simulink model "MS_PID_Control_model"  (R2023a)
settings: Solver=VariableStepAuto  StartTime=0.0  StopTime=2  RelTol=1e-3
values from neighbouring files (symbols this model uses):
  A = [0      1       0           0 ... (first row only)    [MS_PID_Control.m]    (also in SS_PID_Control.m = [0 1;-k/m -c/m])
  amp = 0.01    [MS_PID_Control.m]    (also in SS_PID_Control.m)
  B = [0 k_m/m1 0 -k_m/m2]'    [MS_PID_Control.m]    (also in SS_PID_Control.m = [0;k_f/m])
  C = [-k1/m1 -c1/m1   k1/m1       c1/m1 ... (first row only)    [MS_PID_Control.m]    (also in SS_PID_Control.m = [1 0])
  D = 0    [MS_PID_Control.m]    (also in SS_PID_Control.m)
  den = [L R_m]    [MS_PID_Control.m]
  E = [0 0 0 c2/m2 ... (first row only)    [MS_PID_Control.m]    (also in SS_PID_Control.m = [0 0;c/m k/m])
  Kd = 00070    (= 70)    [MS_PID_Control.m]    (also in SS_PID_Control.m)
  Ki = 13000    [MS_PID_Control.m]    (also in SS_PID_Control.m)
  Kp = 27000    [MS_PID_Control.m]    (also in SS_PID_Control.m)
  num = 1    [MS_PID_Control.m]
libraries: slpidlib x1
settings Model: Creator=z'k'x  LastModifiedBy=z'k'x

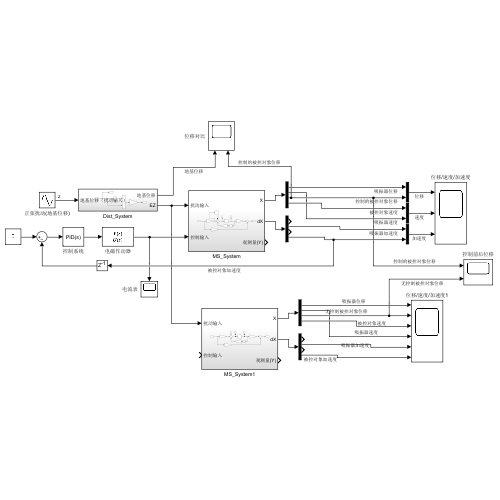
[thumbnail: Simulink's stored preview of the top-level diagram]
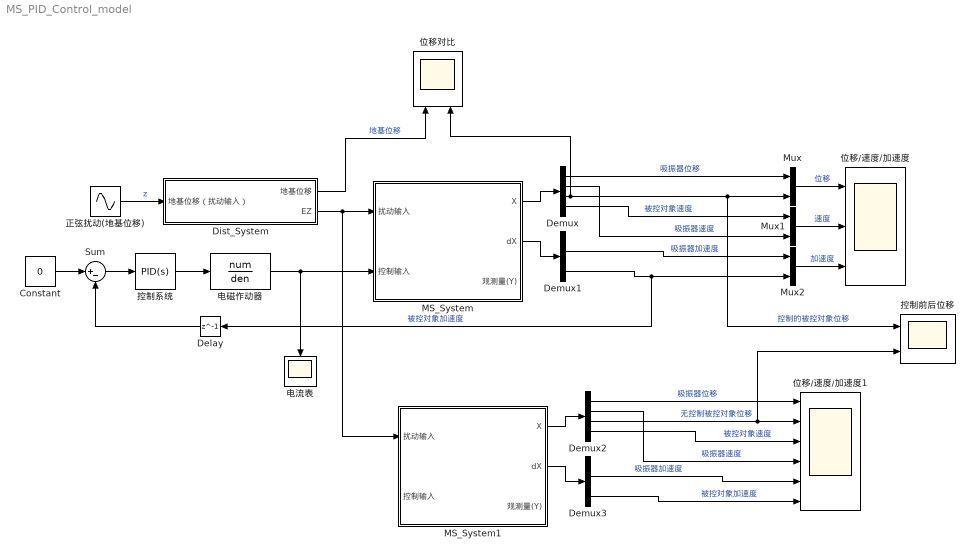
== system MS_PID_Control_model ==
  Constant : Constant  Value=0
  Delay : Delay  DelayLength=1  InitialCondition=0
  Demux{,1..3} (4 alike) : Demux
  Dist_System : Subsystem
  MS_System : Subsystem
  MS_System1 : Subsystem
  Mux : Mux  Inputs=2
  Mux1 : Mux  Inputs=2
  Mux2 : Mux  Inputs=2
  Sum : Sum  Inputs=|+-
  位移/速度/加速度 : Scope  NumInputPorts=3
  位移/速度/加速度1 : Scope  NumInputPorts=6
  位移对比 : Scope  NumInputPorts=2
  控制前后位移 : Scope  NumInputPorts=2
  控制系统 : slpidlib/PID Controller  Controller=PID  Form=Parallel  TimeDomain=Continuous-time  UseExternalTs=off  SampleTime=-1  IntegratorMethod=Forward Euler  FilterMethod=Forward Euler  ControllerParametersSource=internal  P=Kp  I=Ki  UseKiTs=off  D=Kd  N=100  UseFilter=on  TunerSelectOption=Transfer Function Based (PID Tuner App)  InitialConditionSource=internal  InitialConditionForIntegrator=0  InitialConditionForFilter=0  DifferentiatorICPrevScaledInput=0  ExternalReset=none  TrackingMode=off  Kt=1  LimitOutput=off  SatLimitsSource=internal  UpperSaturationLimit=inf  LowerSaturationLimit=-inf  LinearizeAsGain=on  AntiWindupMode=none  Kb=1  LimitIntegrator=off  UpperIntegratorSaturationLimit=inf  LowerIntegratorSaturationLimit=-inf  POutMin=[]  POutMax=[]  IOutMin=[]  IOutMax=[]  DOutMin=[]  DOutMax=[]  NOutMin=[]  NOutMax=[]  SumOutMin=[]  SumOutMax=[]  SaturationOutMin=[]  SaturationOutMax=[]  PParamMin=[]  PParamMax=[]  IParamMin=[]  IParamMax=[]  DParamMin=[]  DParamMax=[]  NParamMin=[]  NParamMax=[]  KbParamMin=[]  KbParamMax=[]  KtParamMin=[]  KtParamMax=[]  KbOutMin=[]  KbOutMax=[]  KtOutMin=[]  KtOutMax=[]  IntegratorOutMin=[]  IntegratorOutMax=[]  FilterOutMin=[]  FilterOutMax=[]  SumI1OutMin=[]  SumI1OutMax=[]  SumI2OutMin=[]  SumI2OutMax=[]  SumI3OutMin=[]  SumI3OutMax=[]  SumI4OutMin=[]  SumI4OutMax=[]  SumDOutMin=[]  SumDOutMax=[]  DifferentiatorOutMin=[]  DifferentiatorOutMax=[]  FilterDiffOutCoefMin=[]  FilterDiffOutCoefMax=[]  ReciprocalOutMin=[]  ReciprocalOutMax=[]  SumDenOutMin=[]  SumDenOutMax=[]  SumNumOutMin=[]  SumNumOutMax=[]  DivideOutMin=[]  DivideOutMax=[]  UdiffTsProdOutMin=[]  UdiffTsProdOutMax=[]  NTsProdOutMin=[]  NTsProdOutMax=[]  UintegralTsProdOutMin=[]  UintegralTsProdOutMax=[]  UngainTsProdOutMin=[]  UngainTsProdOutMax=[]  ClampingZeroOutDataTypeStr=Inherit: Inherit via back propagation  ClampingZeroOutMin=[]  ClampingZeroOutMax=[]  FilterDenConstantOutDataTypeStr=Inherit: Inherit via back propagation  FilterDenConstantOutMin=[]  FilterDenConstantOutMax=[]  PCopyOutDataTypeStr=Inherit: Inherit via back propagation  PCopyOutMin=[]  PCopyOutMax=[]  NCopyOutDataTypeStr=Inherit: Inherit via back propagation  NCopyOutMin=[]  NCopyOutMax=[]  IntegratorContinuousStateAttributes=''  IntegratorStateMustResolveToSignalObject=off  IntegratorRTWStateStorageClass=Auto  FilterContinuousStateAttributes=''  FilterStateMustResolveToSignalObject=off  FilterRTWStateStorageClass=Auto  ParallelPVariant=InternalParameters  IdealPVariant=Disabled  IVariant=InternalParameters  DVariant=InternalParameters  IntegratorVariant=Continuous  SatVariant=Disabled  AWVariant=Passthrough  PCopyVariant=Disabled  TRVariant=Disabled  FdbkBlocksVariant=Forward  IdealPFdbkVariant=Disabled  SatFdbkVariant=Disabled  DerivativeFilterVariant=ContFilter  NVariant=InternalParameters  NCopyVariant=Disabled  FilterICVariant=InternalICsFilter  IntegratorICVariant=InternalICs  ExternalResetVariant=Disabled  TRSumVariant=Passthrough  SumFdbkVariant=Disabled  SumVariant=Sum_PID  TsampFilterVariant=InternalTs  TsampNgainVariant=Passthrough  TsampIntegralVariant=Disabled_SignalSpec  ExternalSaturationOutDataTypeStr=Inherit: Same as second input
  正弦扰动(地基位移) : Sin  Amplitude=amp  Frequency=60*pi  SampleTime=0
  电流表 : Scope
  电磁作动器 : TransferFcn  Numerator=num  Denominator=den
  wires:
  控制系统/1 -> 电磁作动器/1
  正弦扰动(地基位移)/1 -> Dist_System/1(地基位移（扰动输入）)  "z"
  Dist_System/2(EZ) -> MS_System1/1(扰动输入), MS_System/1(扰动输入)
  Dist_System/1(地基位移) -> 位移对比/1  "地基位移"
  MS_System/1(X) -> Demux/1
  MS_System/2(dX) -> Demux1/1
  Demux/1 -> Mux/1  "吸振器位移"
  Demux/4 -> Mux1/1  "被控对象速度"
  Demux/3 -> 位移对比/2, 控制前后位移/1, Mux/2  "控制的被控对象位移"
  Demux/2 -> Mux1/2  "吸振器速度"
  Demux1/2 -> Mux2/1  "吸振器加速度"
  Demux1/4 -> Delay/1, Mux2/2  "被控对象加速度"
  Sum/1 -> 控制系统/1
  Constant/1 -> Sum/1
  Demux3/4 -> 位移/速度/加速度1/6  "被控对象加速度"
  Demux2/3 -> 控制前后位移/2, 位移/速度/加速度1/2  "无控制被控对象位移"
  MS_System1/1(X) -> Demux2/1
  Demux2/4 -> 位移/速度/加速度1/3  "被控对象速度"
  MS_System1/2(dX) -> Demux3/1
  Demux2/2 -> 位移/速度/加速度1/4  "吸振器速度"
  Demux2/1 -> 位移/速度/加速度1/1  "吸振器位移"
  Demux3/2 -> 位移/速度/加速度1/5  "吸振器加速度"
  电磁作动器/1 -> 电流表/1, MS_System/2(控制输入)
  Mux/1 -> 位移/速度/加速度/1  "位移"
  Mux1/1 -> 位移/速度/加速度/2  "速度"
  Mux2/1 -> 位移/速度/加速度/3  "加速度"
  Delay/1 -> Sum/2

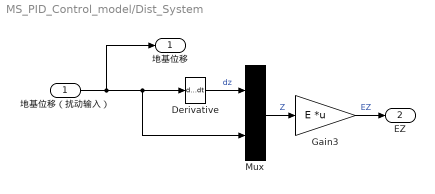
== system MS_PID_Control_model/Dist_System ==
  地基位移（扰动输入） : Inport
  Derivative : Derivative
  Gain3 : Gain  Gain=E  Multiplication=Matrix(K*u) (u vector)
  Mux : Mux  Inputs=2
      settings: DisplayOption=signals
  地基位移 : Outport
  EZ : Outport  Port=2
  wires:
  Gain3/1 -> EZ/1  "EZ"
  Mux/1 -> Gain3/1  "Z"
  Derivative/1 -> Mux/1  "dz"
  地基位移（扰动输入）/1 -> 地基位移/1, Derivative/1, Mux/2

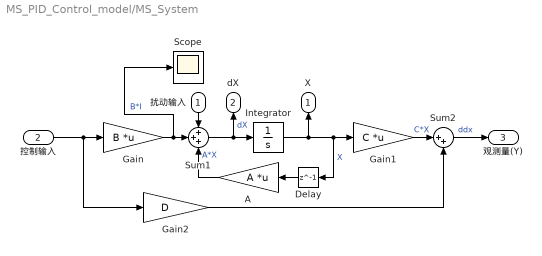
== system MS_PID_Control_model/MS_System ==
  扰动输入 : Inport
  控制输入 : Inport  Port=2
  A : Gain  Gain=A  Multiplication=Matrix(K*u) (u vector)
  Delay : Delay  DelayLength=1  InitialCondition=0
  Gain : Gain  Gain=B  Multiplication=Matrix(K*u) (u vector)
  Gain1 : Gain  Gain=C  Multiplication=Matrix(K*u) (u vector)
  Gain2 : Gain  Gain=D
  Integrator : Integrator
  Scope : Scope
  Sum1 : Sum  Inputs=+++
  Sum2 : Sum  Inputs=|++
  X : Outport
  dX : Outport  Port=2
  观测量(Y) : Outport  Port=3
  wires:
  Gain2/1 -> Sum2/2
  Integrator/1 -> Delay/1, Gain1/1, X/1  "X"
  Sum1/1 -> dX/1, Integrator/1  "dX"
  Gain/1 -> Scope/1, Sum1/2  "B*I"
  Gain1/1 -> Sum2/1  "C*X"
  A/1 -> Sum1/3  "A*X"
  Sum2/1 -> 观测量(Y)/1  "ddx"
  控制输入/1 -> Gain2/1, Gain/1
  扰动输入/1 -> Sum1/1
  Delay/1 -> A/1

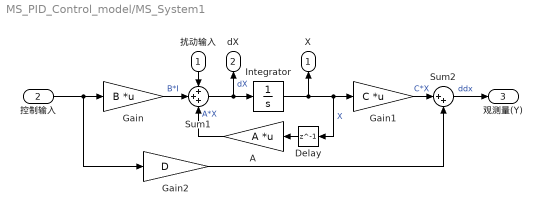
== system MS_PID_Control_model/MS_System1 ==
  扰动输入 : Inport
  控制输入 : Inport  Port=2
  A : Gain  Gain=A  Multiplication=Matrix(K*u) (u vector)
  Delay : Delay  DelayLength=1  InitialCondition=0
  Gain : Gain  Gain=B  Multiplication=Matrix(K*u) (u vector)
  Gain1 : Gain  Gain=C  Multiplication=Matrix(K*u) (u vector)
  Gain2 : Gain  Gain=D
  Integrator : Integrator
  Sum1 : Sum  Inputs=+++
  Sum2 : Sum  Inputs=|++
  X : Outport
  dX : Outport  Port=2
  观测量(Y) : Outport  Port=3
  wires:
  Gain2/1 -> Sum2/2
  Integrator/1 -> Delay/1, Gain1/1, X/1  "X"
  Sum1/1 -> dX/1, Integrator/1  "dX"
  Gain/1 -> Sum1/2  "B*I"
  Gain1/1 -> Sum2/1  "C*X"
  A/1 -> Sum1/3  "A*X"
  Sum2/1 -> 观测量(Y)/1  "ddx"
  控制输入/1 -> Gain2/1, Gain/1
  扰动输入/1 -> Sum1/1
  Delay/1 -> A/1
